simulink model "State_Space_Identifier_Ex8"  (R2023a)
settings: Solver=VariableStepAuto  StartTime=0.0  StopTime=100.0  RelTol=1e-3
undefined symbols (not defined in the file): A, Am, B
libraries: matrix_library x2
settings Model: Creator=geokr  LastModifiedBy=geokr

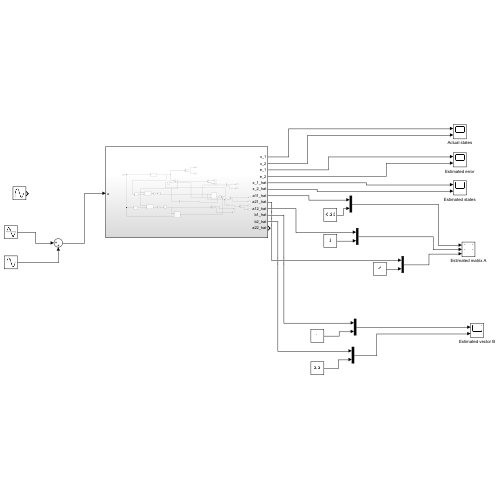
[thumbnail: Simulink's stored preview of the top-level diagram]
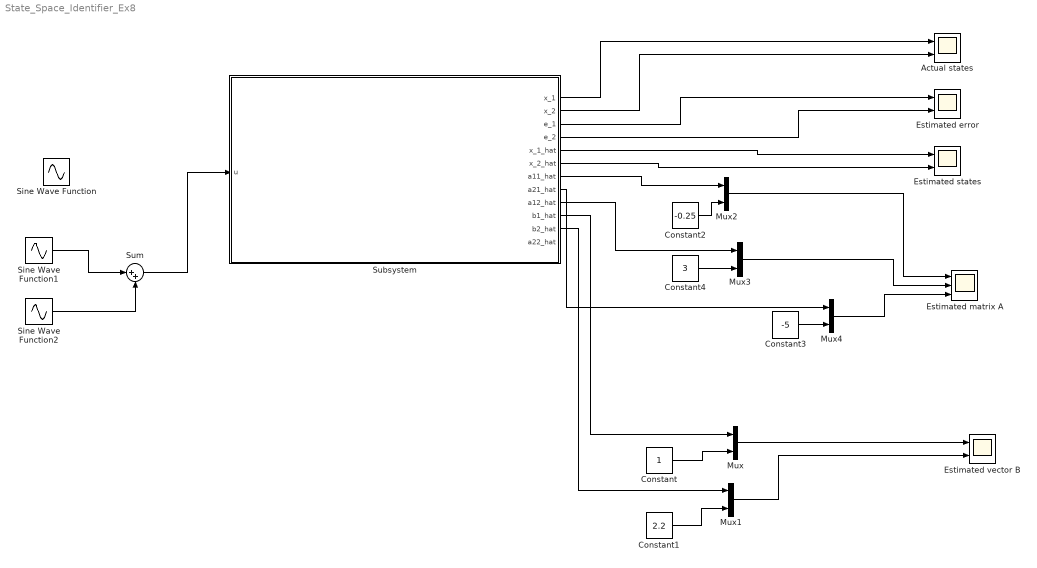
== system State_Space_Identifier_Ex8 ==
  Actual states : Scope  NumInputPorts=2
  Constant : Constant
  Constant1 : Constant  Value=2.2
  Constant2 : Constant  Value=-0.25
  Constant3 : Constant  Value=-5
  Constant4 : Constant  Value=3
  Estimated error : Scope  NumInputPorts=2
  Estimated matrix A : Scope  NumInputPorts=3
  Estimated states : Scope  NumInputPorts=2
  Estimated vector B : Scope  NumInputPorts=2
  Mux{,1..4} (5 alike) : Mux  Inputs=2
  Sine Wave Function : Sin  Amplitude=10  Frequency=2  SampleTime=0
  Sine Wave Function1 : Sin  Amplitude=10  Frequency=2  SampleTime=0
  Sine Wave Function2 : Sin  Amplitude=7  Frequency=3.6  Phase=pi/2  SampleTime=0
  Subsystem : Subsystem
  Sum : Sum  Inputs=|++
  wires:
  Subsystem/1(x_1) -> Actual states/1
  Subsystem/2(x_2) -> Actual states/2
  Subsystem/3(e_1) -> Estimated error/1
  Subsystem/4(e_2) -> Estimated error/2
  Subsystem/5(x_1_hat) -> Estimated states/1
  Subsystem/6(x_2_hat) -> Estimated states/2
  Subsystem/10(b1_hat) -> Mux/1
  Constant/1 -> Mux/2
  Subsystem/11(b2_hat) -> Mux1/1
  Constant1/1 -> Mux1/2
  Mux/1 -> Estimated vector B/1
  Mux1/1 -> Estimated vector B/2
  Mux2/1 -> Estimated matrix A/1
  Mux3/1 -> Estimated matrix A/2
  Subsystem/7(a11_hat) -> Mux2/1
  Constant2/1 -> Mux2/2
  Constant4/1 -> Mux3/2
  Constant3/1 -> Mux4/2
  Subsystem/8(a21_hat) -> Mux4/1
  Subsystem/9(a12_hat) -> Mux3/1
  Sine Wave Function1/1 -> Sum/1
  Sine Wave Function2/1 -> Sum/2
  Mux4/1 -> Estimated matrix A/3
  Sum/1 -> Subsystem/1(u)

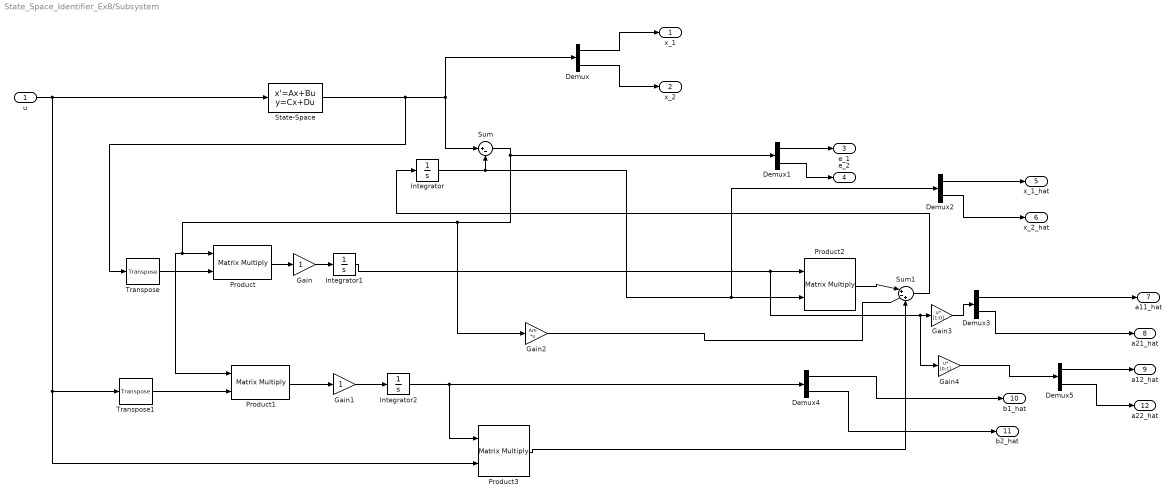
== system State_Space_Identifier_Ex8/Subsystem ==
  u : Inport
  Demux{,1..5} (6 alike) : Demux  Outputs=2
  Gain : Gain
  Gain1 : Gain
  Gain2 : Gain  Gain=Am  Multiplication=Matrix(K*u)
  Gain3 : Gain  Gain=[1;0]  Multiplication=Matrix(u*K)
  Gain4 : Gain  Gain=[0;1]  Multiplication=Matrix(u*K)
  Integrator : Integrator
  Integrator1 : Integrator
  Integrator2 : Integrator
  Product{,1..3} (4 alike) : Product  Multiplication=Matrix(*)
  State-Space : StateSpace  A=A  B=B  C=[1 0;0 1]  D=[0;0]  InitialCondition=[0,0]
  Sum : Sum  Inputs=|+-
  Sum1 : Sum  Inputs=|+-+
  Transpose : matrix_library/Transpose
  Transpose1 : matrix_library/Transpose
  x_1 : Outport
  x_2 : Outport  Port=2
  e_1 : Outport  Port=3
  e_2 : Outport  Port=4
  x_1_hat : Outport  Port=5
  x_2_hat : Outport  Port=6
  a11_hat : Outport  Port=7
  a21_hat : Outport  Port=8
  a12_hat : Outport  Port=9
  b1_hat : Outport  Port=10
  b2_hat : Outport  Port=11
  a22_hat : Outport  Port=12
  wires:
  Gain1/1 -> Integrator2/1
  u/1 -> State-Space/1, Transpose1/1, Product3/2
  State-Space/1 -> Demux/1, Sum/1, Transpose/1
  Sum/1 -> Demux1/1, Gain2/1, Product/1, Product1/1
  Integrator/1 -> Product2/2, Demux2/1, Sum/2
  Gain/1 -> Integrator1/1
  Product3/1 -> Sum1/3
  Transpose/1 -> Product/2
  Transpose1/1 -> Product1/2
  Integrator2/1 -> Demux4/1, Product3/1
  Product/1 -> Gain/1
  Gain2/1 -> Sum1/2
  Demux/2 -> x_2/1
  Product1/1 -> Gain1/1
  Product2/1 -> Sum1/1
  Integrator1/1 -> Product2/1, Gain4/1, Gain3/1
  Sum1/1 -> Integrator/1
  Demux/1 -> x_1/1
  Demux1/1 -> e_1/1
  Demux1/2 -> e_2/1
  Demux2/1 -> x_1_hat/1
  Demux2/2 -> x_2_hat/1
  Demux3/1 -> a11_hat/1
  Demux3/2 -> a21_hat/1
  Demux4/1 -> b1_hat/1
  Demux4/2 -> b2_hat/1
  Gain3/1 -> Demux3/1
  Demux5/1 -> a12_hat/1
  Gain4/1 -> Demux5/1
  Demux5/2 -> a22_hat/1
